simulink model "Plant_2_1"  (R2024b)
settings: Solver=FixedStepAuto  StartTime=0.0  StopTime=20  FixedStep=0.02  RelTol=1e-3
values from neighbouring files (symbols this model uses):
  A = zeros(4, 4)    [Initialise_var_0.m]
  B = zeros(4, 2)    [Initialise_var_0.m]
  C = [1 0 0 0; 0 1 0 0]    [Initialise_var_0.m]    (also in leunberger_obs_1.m; sfbia.m)
  D = [0 0; 0 0]    [Initialise_var_0.m]    (also in leunberger_obs_1.m = [0 0;0 0]; sfbia.m = [0 0;0 0])
  K = place(A, B, desired_poles)    [leunberger_obs_1.m]    (also in state_feedback.m; state_feedback_0.m; state_feedback_3.m; state_feedback_4.m = lqr(A,B,Q,R))
  L1 = 0.095    [Initialise_var_0.m]
  L2 = 0.095    [Initialise_var_0.m]
settings Model: Creator=Sez26  LastModifiedBy=Sez26

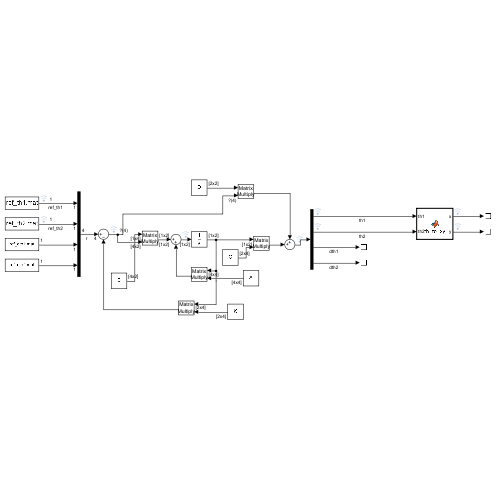
[thumbnail: Simulink's stored preview of the top-level diagram]
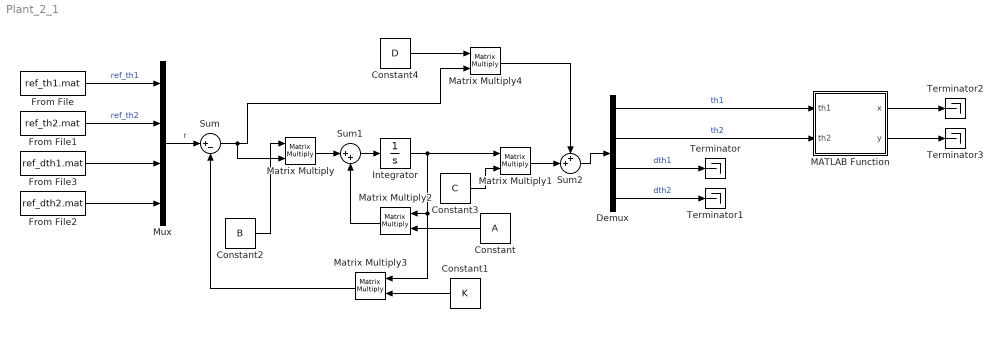
== system Plant_2_1 ==
  Constant : Constant  Value=A
  Constant1 : Constant  Value=K
  Constant2 : Constant  Value=B
  Constant3 : Constant  Value=C
  Constant4 : Constant  Value=D
  Demux : Demux
  From File : FromFile  FileName=ref_th1.mat  SampleTime=0
  From File1 : FromFile  FileName=ref_th2.mat  SampleTime=0
  From File2 : FromFile  FileName=ref_dth2.mat  SampleTime=0
  From File3 : FromFile  FileName=ref_dth1.mat  SampleTime=0
  Integrator : Integrator
  MATLAB Function : MATLAB Function  TreatAsAtomicUnit=on
  Matrix Multiply{,1..4} (5 alike) : Product  Multiplication=Matrix(*)
  Mux : Mux
  Sum : Sum  Inputs=|+-
  Sum1 : Sum  Inputs=|++
  Sum2 : Sum  Inputs=++|
  Terminator{,1..3} (4 alike) : Terminator
  wires:
  MATLAB Function/1(x) -> Terminator2/1
  MATLAB Function/2(y) -> Terminator3/1
  From File3/1 -> Mux/3
  From File2/1 -> Mux/4
  From File/1 -> Mux/1  "ref_th1"
  From File1/1 -> Mux/2  "ref_th2"
  Demux/3 -> Terminator/1  "dth1"
  Demux/4 -> Terminator1/1  "dth2"
  Demux/2 -> MATLAB Function/2(th2)  "th2"
  Demux/1 -> MATLAB Function/1(th1)  "th1"
  Mux/1 -> Sum/1  "r"
  Sum/1 -> Matrix Multiply/2, Matrix Multiply4/2
  Matrix Multiply/1 -> Sum1/1
  Sum1/1 -> Integrator/1
  Integrator/1 -> Matrix Multiply3/1, Matrix Multiply2/1, Matrix Multiply1/1
  Constant3/1 -> Matrix Multiply1/2
  Matrix Multiply1/1 -> Sum2/2
  Sum2/1 -> Demux/1
  Constant/1 -> Matrix Multiply2/2
  Matrix Multiply2/1 -> Sum1/2
  Constant1/1 -> Matrix Multiply3/2
  Matrix Multiply3/1 -> Sum/2
  Constant4/1 -> Matrix Multiply4/1
  Matrix Multiply4/1 -> Sum2/1
  Constant2/1 -> Matrix Multiply/1

== matlab function Plant_2_1/MATLAB Function ==
  data: x output; th1 input; y output; th2 input; L1 parameter; L2 parameter
function [x,y] = th_to_xy(th1, th2, L1, L2)
    x = L1*cos(deg2rad(th1)) + L2*cos(deg2rad(th2));
    y = L1*sin(deg2rad(th1)) + L2*sin(deg2rad(th2));
